simulink library "DBX_model"  (R2015a)
settings: Solver=ode45  SolverMode=SingleTasking  StartTime=0.0  StopTime=10.0  RelTol=1e-3
undefined symbols (not defined in the file): a, A_M, Activo, C_d0, Ganancia, h, h_1, h_3, Initial_Omegas, Initial_Torques, J_T, kappa_Q, kappa_T, l, L_M, lambda_0_Q, lambda_0_T, Motor, Newton, Prop, R, Raphson, rho, Rotation_sign, sigma, Tau_motors, theta_0, theta_1, Throtle_TTO_vec, Torque_TTO_vec, trim_control, v_i0, v_i_adim, Vx_adim, Vz_adim
libraries: vrlib x11, DBX_model x9, simulink x3, aerolibutil x3, dspinverses x1
settings Model: Creator=David  LastModifiedBy=david
settings OptimizationCC: BlockReduction=off  BooleanDataType=off
settings DebuggingCC: SaveWithParameterizedLinksMsg=none  UnderspecifiedInitializationDetection=Classic  MergeDetectMultiDrivingBlocksExec=none  SignalResolutionControl=TryResolveAllWithWarning  StrictBusMsg=Warning
settings HardwareCC: TargetUnknown=on

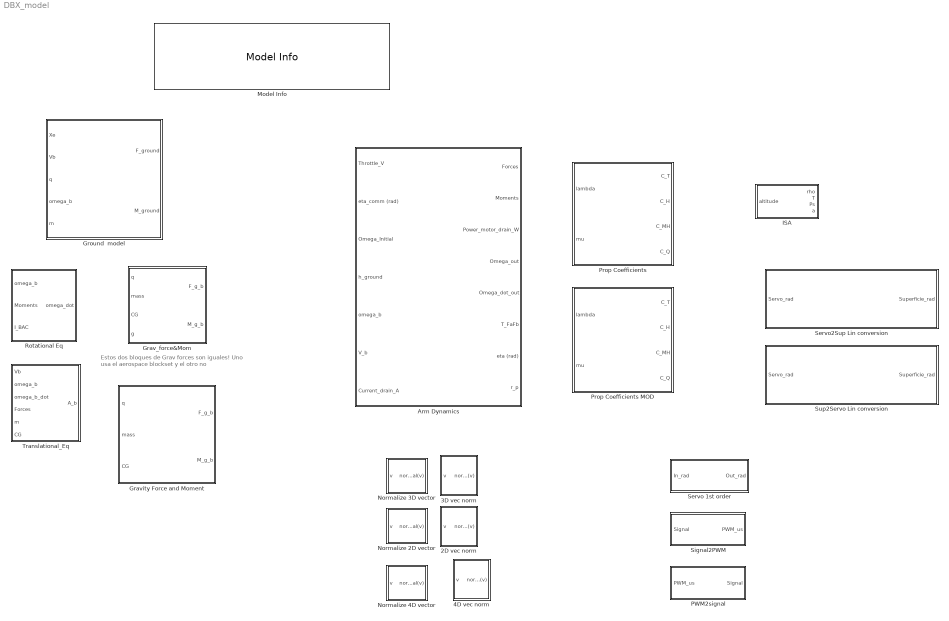
== system DBX_model ==
  note: Estos dos bloques de Grav forces son iguales!
      | Uno usa el aerospace blockset y el otro no
  2D vec norm : Subsystem
  3D vec norm : Subsystem
  4D vec norm : Subsystem
  Arm Dynamics : Subsystem  mask(Arm dynamics, kinematics, forces and moments){arm_num=1, Rot_sign=Rotation_sign(1), Hub_pos=l*[1;0;0], h_p=h, Gain=[1;0;0], UpperLimit=deg2rad(10), LowerLimit=-deg2rad(100), J_FA=0, Inertia_swithc_var=Motor+Prop, Freno_param=Activo, J_T=J_T, tau=Tau_motors, Initi_omega=Initial_Omegas(1), Init_torque=Initial_Torques(1), omega_n=35, xi=1.45, init_eta=0, Gain_servos=1, Bias=0.0}
      mask prompts: arm_num "Arm number (1,2 or 3)"; Rot_sign "Rotation sign"; Hub_pos "Hub position"; h_p "Hub to porpeller dist"; Gain "eta dir"; UpperLimit "eta sup lim"; LowerLimit "eta inf lim"; J_FA "J Fore arm"; Inertia_swithc_var "Which inertia to use?"; Freno_param "Freando o Activo"; J_T "Inertia Motor+Prop"; tau "Tau motors"; Initi_omega "Initial Omega (rad/s)"; Init_torque "Initial Torque(Nm)"; omega_n "Servo natural freq (rad/s) omega_n"; xi "Servo damping xi"; init_eta "Initial eta_servo (rad)"; Gain_servos "Pendiente Sup_rad/Servo_rad"; Bias "Sup_rad_0: Deflexion superficie con servo en 1500us"
      mask help:
      | This block only accepts arms oriented in x-axis or y-axis: eta direction can only be [1,0,0] or [0,1,0]
      |
      | If Arm number 1 or  2 (Forward ones)
      | eta_dir==[0,1,0]
      |
      | If Arm number 3 (rear one)
      | eta_dir=[1,0,0]
      |
      | Usar SIEMPRE SI
      mask TypeOptions arm_num: Arms Kinematics DBX/Value
      mask TypeOptions Rot_sign: Gyroscopic Moments DBX/Rot_sign | Aerodynamics Propeller DBX/Rot_signa
      mask TypeOptions Hub_pos: Arms Kinematics DBX/Hub_pos
      mask TypeOptions h_p: Arms Kinematics DBX/h_p
      mask TypeOptions Gain: Arms Kinematics DBX/Gain | Gyroscopic Moments DBX/Gain
      mask TypeOptions UpperLimit: Servos Dynamics DBX/UpperLimit
      mask TypeOptions LowerLimit: Servos Dynamics DBX/LowerLimit
      mask TypeOptions J_FA: Gyroscopic Moments DBX/J_FA
      mask TypeOptions Inertia_swithc_var: ESC+Motor Dynamcis DBX/Inertia_swithc_var
      mask TypeOptions Freno_param: ESC+Motor Dynamcis DBX/Freno_param
      mask TypeOptions J_T: ESC+Motor Dynamcis DBX/J_T | Gyroscopic Moments DBX/J_T
      mask TypeOptions tau: ESC+Motor Dynamcis DBX/tau
      mask TypeOptions Initi_omega: initial_omega/X0
      mask TypeOptions Init_torque: Initial_torque/X0
      mask TypeOptions omega_n: Servos Dynamics DBX/omega_n
      mask TypeOptions xi: Servos Dynamics DBX/xi | Servos Dynamics DBX/derv_param
      mask TypeOptions init_eta: Servos Dynamics DBX/init_eta
      mask TypeOptions Gain_servos: Servo2Sup Lin conversion/Gain
      mask TypeOptions Bias: Servo2Sup Lin conversion/Bias
      mask Display: disp(['{\bf \fontsize{16}',sprintf('Arm number\n\n'),num2str(arm_num),sprintf('\n\n Dynamics '),'}'], 'texmode','on');
  Grav_force&Mom : Subsystem
  Gravity Force and Moment : MATLAB Function
  Ground  model : Subsystem
  ISA : MATLAB Function  TreatAsAtomicUnit=on
  Model Info : simulink/Model-Wide Utilities/Model Info  Frame=on  DisplayStringWithTags=|  HorizontalTextAlignment=Center  LeftAlignmentValue=0.5  SourceBlockDiagram=DBX_model  TagMaxNumber=20
      | Model Info
      | 
      | Creado por %<Creator>
      | Modificado el %<LastModificationDate> por %<LastModifiedBy>
      | Version %<ModelVersion>
  Normalize 2D vector : Subsystem
  Normalize 3D vector : Subsystem
  Normalize 4D vector : Subsystem
  PWM2signal : Subsystem  TreatAsAtomicUnit=on  mask{c=1900, a=1100, d=1, b=0}
      mask prompts: c "PWM sup limit (us)"; a "PWM inf limit (us)"; d "Signal sup limit"; b "Signal inf limit"
      mask TypeOptions c: up_PWM/Value
      mask TypeOptions a: down_PWM/Value
      mask TypeOptions d: up_signal/Value
      mask TypeOptions b: down_signal/Value
  Prop Coefficients : MATLAB Function
  Prop Coefficients MOD : MATLAB Function
  Rotational Eq : Subsystem
  Servo 1st order : Subsystem  TreatAsAtomicUnit=on  mask{Init_def=0, Max_rate=6.159, Min_rate=-6.159, Max_defle=deg2rad(25), Min_def=-deg2rad(25), RT=0.01}
      mask prompts: Init_def "Initial deflection (rad)"; Max_rate "Maximo rate (rad/s)"; Min_rate "Minimo rate (rad/s)"; Max_defle "Maxima deflexion (rad)"; Min_def "Minima deflexion (rad)"; RT "Rise Time"
      mask TypeOptions Init_def: Initial/Value
      mask TypeOptions Max_rate:
      | Rate
      | Saturation/UpperLimit
      mask TypeOptions Min_rate:
      | Rate
      | Saturation/LowerLimit
      mask TypeOptions Max_defle:
      | Command
      | Saturation/UpperLimit | Integrator
      | /UpperSaturationLimit
      mask TypeOptions Min_def:
      | Command
      | Saturation/LowerLimit | Integrator
      | /LowerSaturationLimit
      mask Callback RT:
      | vals=get_param(gcb,'MaskValues');
      | Ganancia = 1/str2num(vals{6});
  Servo2Sup Lin conversion : Subsystem  mask{Gain=1, Bias=0.0}
      mask prompts: Gain "Pendiente Sup_rad/Servo_rad"; Bias "Sup_rad_0: Deflexion superficie con servo en 1500us"
      mask TypeOptions Gain: Gain/Gain
      mask TypeOptions Bias: Bias/Bias
      mask DialogControl DescTextVar Prompt: Conversion de roation del servo en rad a deflexion de las superficie de control en rad. Usar la funcion de matlab para encontrar las variables de abajo
      mask Display:
      | x=-pi:0.1:pi;
      | y=Gain.*x+Bias;
      | 
      | plot(x,y);
      | 
      | 
      | port_label('output', 1, 'Defl Superficie rad')
      | 
      | port_label('input', 1, 'Rotacion servo rad')
  Signal2PWM : Subsystem  TreatAsAtomicUnit=on  mask{b=1, d=0, a=1900, c=1100}
      mask prompts: b "Signal sup limit"; d "Signal inf limit"; a "PWM sup limit (us)"; c "PWM inf limit (us)"
      mask TypeOptions b: up_signal/Value
      mask TypeOptions d: down_signal/Value
      mask TypeOptions a: up_PWM/Value
      mask TypeOptions c: down_PWM/Value
  Sup2Servo Lin conversion : Subsystem  mask{Gain=1, Bias=0.0}
      mask prompts: Gain "Pendiente Sup_rad/Servo_rad"; Bias "Sup_rad_0: Deflexion superficie con servo en 1500us"
      mask TypeOptions Gain: Sup to servo pendiente/Value
      mask TypeOptions Bias: Sup_0_rad/Value
      mask DialogControl DescTextVar Prompt: Conversion de deflexion de la superficie en rad a rotacion del servo en rad. Usar la funcion de matlab para encontrar las variables de abajo
      mask Display:
      | x=-pi:0.1:pi;
      | y=(x-Bias)./Gain;
      | 
      | plot(x,y);
      | 
      | port_label('output', 1, 'Rotacion servo rad')
      | port_label('input', 1, 'Defl Superficie rad')
  Translational_Eq : Subsystem

== system DBX_model/2D vec norm ==
  v : Inport
  norm^2rm : Subsystem  TreatAsAtomicUnit=on
  sqrt : Sqrt  AlgorithmType=Newton-Raphson  SaturateOnIntegerOverflow=on
  norm(v) : Outport
  wires:
  sqrt/1 -> norm(v)/1
  norm^2rm/1(norm(v)) -> sqrt/1
  v/1 -> norm^2rm/1(v)

== system DBX_model/3D vec norm ==
  v : Inport
  norm^2rm : Subsystem  TreatAsAtomicUnit=on
  sqrt : Sqrt  AlgorithmType=Newton-Raphson  SaturateOnIntegerOverflow=on
  norm(v) : Outport
  wires:
  v/1 -> norm^2rm/1(v)
  norm^2rm/1(norm(v)) -> sqrt/1
  sqrt/1 -> norm(v)/1

== system DBX_model/4D vec norm ==
  v : Inport
  norm^2rm : Subsystem  TreatAsAtomicUnit=on
  sqrt : Sqrt  AlgorithmType=Newton-Raphson  SaturateOnIntegerOverflow=on
  norm(v) : Outport
  wires:
  sqrt/1 -> norm(v)/1
  norm^2rm/1(norm(v)) -> sqrt/1
  v/1 -> norm^2rm/1(v)

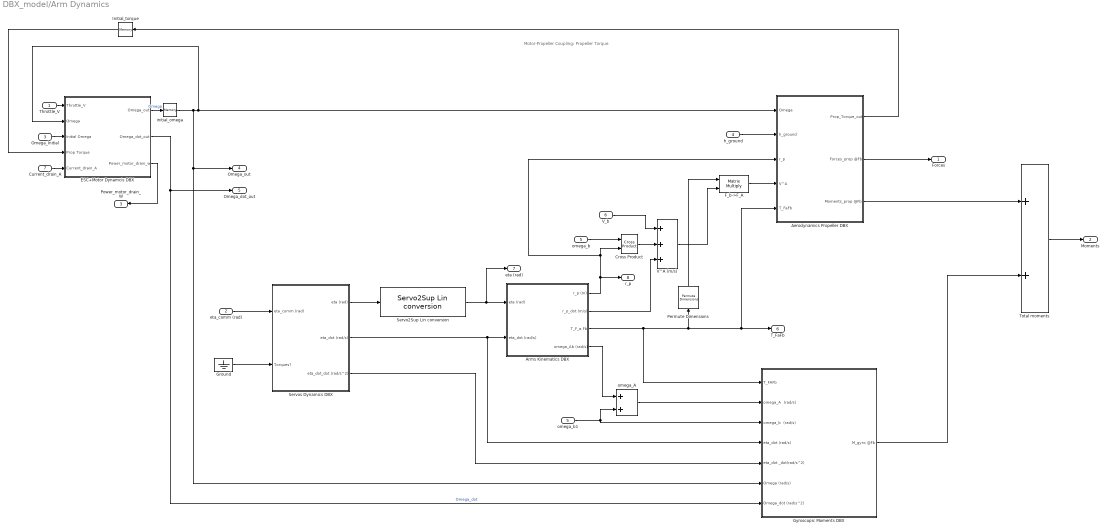
== system DBX_model/Arm Dynamics ==
  note: Motor-Propeller Coupling: Propeller Torque
  Throttle_V : Inport
  eta_comm (rad) : Inport  Port=2
  Omega_Initial : Inport  Port=3
  h_ground : Inport  Port=4
  omega_b : Inport  Port=5
  V_b : Inport  Port=6
  Current_drain_A : Inport  Port=7
  Aerodynamics Propeller DBX : Subsystem  mask{Rot_signa=Rot_sign}
      mask prompts: Rot_signa "Rotation Sign"
      settings: MinAlgLoopOccurrences=on
      mask TypeOptions Rot_signa: Rotation_sign/Value
  Arms Kinematics DBX : Subsystem  mask{Value=arm_num, Hub_pos=Hub_pos, h_p=h_p, Gain=Gain}
      mask prompts: Value "Arm number (1,2 or 3)"; Hub_pos "Hub position"; h_p "Hub to porpeller dist"; Gain "eta dir"
      mask TypeOptions Value: Arm_no/Value
      mask TypeOptions Hub_pos: Hub_position aka r_RP_i/Value
      mask TypeOptions h_p: h_p_i/Value
      mask TypeOptions Gain: eta_dir/Gain
  Cross Product : vrlib/Utilities/Cross Product
  ESC+Motor Dynamcis DBX : Subsystem  mask{Inertia_swithc_var=Motor+Prop, J_T=J_T, tau=tau, Freno_param=Activo}
      mask prompts: Inertia_swithc_var "Which inertia to use?"; J_T "Inertia Motor+Prop"; tau "Tau motors"; Freno_param "Freando o Activo"
      mask init:
      | val = get_param(gcb,'MaskValues');
      | switch lower(val{4})
      |  case {'frenado'}
      |   Freno=0;
      |  case {'activo'}
      |   Freno=1;
      | end
      mask TypeOptions Inertia_swithc_var: None | Motor+Prop
      mask Callback Inertia_swithc_var:
      | val = get_param(gcb,'MaskValues');
      | % lower(val{1})
      | switch lower(val{1})
      |  case {'none'}
      |   inertia_switch=1;
      |  case {'motor+prop'}
      |   inertia_switch=2;
      | end
      mask TypeOptions J_T: Inertia of prop+motor/Value
      mask TypeOptions tau: Time constant motors/Value
      mask TypeOptions Freno_param: Frenado | Activo
      mask Callback Freno_param:
      | val = get_param(gcb,'MaskValues');
      | switch lower(val{4})
      |  case {'frenado'}
      |   Freno=0;
      |  case {'activo'}
      |   Freno=1;
      | end
  F_b->F_A : Product  Multiplication=Matrix(*)
  Ground : Ground
  Gyroscopic Moments DBX : Subsystem  mask{Rot_sign=Rot_sign, Gain=Gain, J_T=J_T, J_FA=J_FA}
      mask prompts: Rot_sign "Rotation sign"; Gain "eta direction"; J_T "Motor&prop inertia"; J_FA "J Fore arm"
      mask TypeOptions Rot_sign: Rotation_sign/Value | Rotation_sign1/Value
      mask TypeOptions Gain: eta_dir/Gain | eta_dir1/Gain
      mask TypeOptions J_T: Propeller and motor inertia1/Value | Propeller and motor inertia/Value
  Initial_torque : Memory  X0=Init_torque  InheritSampleTime=on
  Permute Dimensions : PermuteDimensions
  Servo2Sup Lin conversion : DBX_model/Servo2Sup Lin conversion  Gain=Gain_servos  Bias=Bias
  Servos Dynamics DBX : Subsystem  mask{omega_n=omega_n, xi=xi, derv_param=xi, init_eta=init_eta, UpperLimit=UpperLimit, LowerLimit=LowerLimit, Gain=Gain_servos, Bias=Bias}
      mask prompts: omega_n "Servo natural freq (rad/s) omega_n"; xi "Servo damping xi"; derv_param "Derivative parameter"; init_eta "Initial eta_servo (rad)"; UpperLimit "eta Sup lim"; LowerLimit "eta inf lim"; Gain "Pendiente Sup_rad/Servo_rad"; Bias "Sup_rad_0: Deflexion superficie con servo en 1500us"
      mask TypeOptions init_eta: init_eta/Value | init_eta1/Value
      mask TypeOptions UpperLimit: upper limit/Value
      mask TypeOptions LowerLimit: Lower limit/Value
      mask TypeOptions Gain: Sup2Servo Lin conversion/Gain | Sup2Servo Lin conversion1/Gain
      mask TypeOptions Bias: Sup2Servo Lin conversion/Bias | Sup2Servo Lin conversion1/Bias
  Total moments : Sum
  V^A (m/s) : Sum  Inputs=+++
  initial_omega : Memory  X0=Initi_omega  InheritSampleTime=on
  omega_A : Sum
  omega_b1 : InportShadow  Port=5
  Forces : Outport
  Moments : Outport  Port=2
  Power_motor_drain_W : Outport  Port=3
  Omega_out : Outport  Port=4
  Omega_dot_out : Outport  Port=5
  T_FaFb : Outport  Port=6
  eta (rad) : Outport  Port=7
  r_p : Outport  Port=8
  wires:
  Throttle_V/1 -> ESC+Motor Dynamcis DBX/1(Throttle_V)
  Omega_Initial/1 -> ESC+Motor Dynamcis DBX/3(Initial Omega)
  ESC+Motor Dynamcis DBX/2(Omega_dot_out) -> Gyroscopic Moments DBX/7(Omega_dot (rad/s^2)), Omega_dot_out/1  "Omega_dot"
  ESC+Motor Dynamcis DBX/1(Omega_out) -> initial_omega/1  "Omega"
  h_ground/1 -> Aerodynamics Propeller DBX/2(h_ground)
  Servos Dynamics DBX/1(eta (rad)) -> Servo2Sup Lin conversion/1
  omega_b/1 -> Cross Product/1
  Cross Product/1 -> V^A (m/s)/2
  V_b/1 -> V^A (m/s)/1
  Arms Kinematics DBX/2(r_p_dot (m/s)) -> V^A (m/s)/3
  F_b->F_A/1 -> Aerodynamics Propeller DBX/4(V^A)
  Arms Kinematics DBX/3(T_F_a,Fb) -> Gyroscopic Moments DBX/1(T_FAFb), Permute Dimensions/1, Aerodynamics Propeller DBX/5(T_FaFb), T_FaFb/1
  Arms Kinematics DBX/1(r_p (m)) -> Aerodynamics Propeller DBX/3(r_p), Cross Product/2, r_p/1
  Aerodynamics Propeller DBX/2(Forces_prop @Fb) -> Forces/1
  Servos Dynamics DBX/2(eta_dot (rad/s)) -> Gyroscopic Moments DBX/4(eta_dot (rad/s)), Arms Kinematics DBX/2(eta_dot (rad/s))
  Arms Kinematics DBX/4(omega_Ab (rad/s)) -> omega_A/1
  omega_b1/1 -> Gyroscopic Moments DBX/3(omega_b  (rad/s)), omega_A/2
  omega_A/1 -> Gyroscopic Moments DBX/2(omega_A  (rad/s))
  Servos Dynamics DBX/3(eta_dot_dot (rad/s^2)) -> Gyroscopic Moments DBX/5(eta_dot _dot(rad/s^2))
  Ground/1 -> Servos Dynamics DBX/2(Torques?)
  Aerodynamics Propeller DBX/3(Moments_prop @Fb) -> Total moments/1
  Gyroscopic Moments DBX/1(M_gyro @Fb) -> Total moments/2
  Total moments/1 -> Moments/1
  Aerodynamics Propeller DBX/1(Prop_Torque_out) -> Initial_torque/1
  Initial_torque/1 -> ESC+Motor Dynamcis DBX/4(Prop Torque)
  eta_comm (rad)/1 -> Servos Dynamics DBX/1(eta_comm (rad))
  Servo2Sup Lin conversion/1 -> Arms Kinematics DBX/1(eta (rad)), eta (rad)/1
  V^A (m/s)/1 -> F_b->F_A/2
  Permute Dimensions/1 -> F_b->F_A/1
  initial_omega/1 -> Aerodynamics Propeller DBX/1(Omega), ESC+Motor Dynamcis DBX/2(Omega), Gyroscopic Moments DBX/6(Omega (rad/s)), Omega_out/1
  ESC+Motor Dynamcis DBX/3(Power_motor_drain_w) -> Power_motor_drain_W/1
  Current_drain_A/1 -> ESC+Motor Dynamcis DBX/5(Current_drain_A)

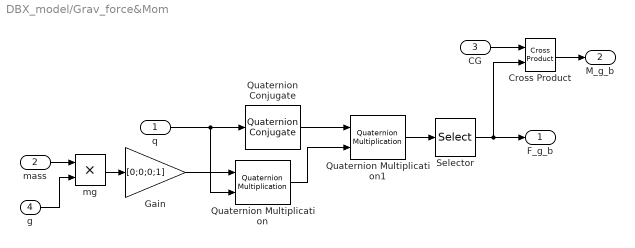
== system DBX_model/Grav_force&Mom ==
  q : Inport
  mass : Inport  Port=2
  CG : Inport  Port=3
  g : Inport  Port=4
  Cross Product : vrlib/Utilities/Cross Product
  Gain : Gain  Gain=[0;0;0;1]
  Quaternion Conjugate : aerolibutil/Quaternion Conjugate
  Quaternion Multiplication : aerolibutil/Quaternion Multiplication
  Quaternion Multiplication1 : aerolibutil/Quaternion Multiplication
  Selector : Selector  IndexMode=Zero-based  InputPortWidth=4  Indices=[1:3]
  mg : Product  RndMeth=Zero
  F_g_b : Outport
  M_g_b : Outport  Port=2
  wires:
  mass/1 -> mg/1
  g/1 -> mg/2
  mg/1 -> Gain/1
  Gain/1 -> Quaternion Multiplication/1
  q/1 -> Quaternion Conjugate/1, Quaternion Multiplication/2
  Quaternion Conjugate/1 -> Quaternion Multiplication1/1
  Quaternion Multiplication/1 -> Quaternion Multiplication1/2
  Quaternion Multiplication1/1 -> Selector/1
  Selector/1 -> Cross Product/2, F_g_b/1
  CG/1 -> Cross Product/1
  Cross Product/1 -> M_g_b/1

== system DBX_model/Ground  model ==
  Xe : Inport
  Vb : Inport  Port=2
  q : Inport  Port=3
  omega_b : Inport  Port=4
  m : Inport  Port=5
  Ground model logic and Forces and moments : MATLAB Function  TreatAsAtomicUnit=on
  arm_hub position 1 : Constant  Value=[1/3*L_M;-A_M/2;h_1]
  arm_hub position 2 : Constant  Value=[1/3*L_M;A_M/2;h_1]
  arm_hub position 3 : Constant  Value=[-2/3*L_M;0;h_3]
  F_ground : Outport
  M_ground : Outport  Port=2
  wires:
  omega_b/1 -> Ground model logic and Forces and moments/4(omega_b)
  Vb/1 -> Ground model logic and Forces and moments/2(Vb)
  Ground model logic and Forces and moments/1(F_gr_b) -> F_ground/1
  Ground model logic and Forces and moments/2(M_gr_b) -> M_ground/1
  arm_hub position 3/1 -> Ground model logic and Forces and moments/8(Arm3)
  arm_hub position 2/1 -> Ground model logic and Forces and moments/7(Arm2)
  arm_hub position 1/1 -> Ground model logic and Forces and moments/6(Arm1)
  m/1 -> Ground model logic and Forces and moments/5(mass)
  q/1 -> Ground model logic and Forces and moments/3(q)
  Xe/1 -> Ground model logic and Forces and moments/1(Xe)

== system DBX_model/Normalize 2D vector ==
  v : Inport
  2D vec norm : DBX_model/2D vec norm
  Bias : Bias  Bias=eps
  Demux : Demux  Outputs=2
  Math Function : Math  Operator=reciprocal  SaturateOnIntegerOverflow=on
  Mux : Mux  Inputs=2
  Product2 : Product  Inputs=**
  Product3 : Product  Inputs=**
  normal(v) : Outport
  wires:
  Math Function/1 -> Product2/2, Product3/2
  Demux/2 -> Product3/1
  Demux/1 -> Product2/1
  Mux/1 -> normal(v)/1
  v/1 -> 2D vec norm/1, Demux/1
  Bias/1 -> Math Function/1
  Product2/1 -> Mux/1
  Product3/1 -> Mux/2
  2D vec norm/1 -> Bias/1

== system DBX_model/Normalize 3D vector ==
  v : Inport
  3D vec norm : DBX_model/3D vec norm
  Bias : Bias  Bias=eps
  Demux : Demux  Outputs=3
  Math Function : Math  Operator=reciprocal  SaturateOnIntegerOverflow=on
  Mux : Mux  Inputs=3
  Product1 : Product  Inputs=**
  Product2 : Product  Inputs=**
  Product3 : Product  Inputs=**
  normal(v) : Outport
  wires:
  Demux/2 -> Product3/1
  Demux/1 -> Product2/1
  Mux/1 -> normal(v)/1
  v/1 -> 3D vec norm/1, Demux/1
  3D vec norm/1 -> Bias/1
  Product2/1 -> Mux/1
  Product3/1 -> Mux/2
  Demux/3 -> Product1/1
  Math Function/1 -> Product2/2, Product3/2, Product1/2
  Product1/1 -> Mux/3
  Bias/1 -> Math Function/1

== system DBX_model/Normalize 4D vector ==
  v : Inport
  4D vec norm : DBX_model/4D vec norm
  Bias : Bias  Bias=eps
  Demux : Demux
  Math Function : Math  Operator=reciprocal  SaturateOnIntegerOverflow=on
  Mux : Mux
  Product{1..4} (4 alike) : Product  Inputs=**
  normal(v) : Outport
  wires:
  Product4/1 -> Mux/4
  Demux/4 -> Product4/1
  Demux/2 -> Product3/1
  Demux/1 -> Product2/1
  Mux/1 -> normal(v)/1
  v/1 -> 4D vec norm/1, Demux/1
  4D vec norm/1 -> Bias/1
  Product2/1 -> Mux/1
  Product3/1 -> Mux/2
  Demux/3 -> Product1/1
  Math Function/1 -> Product2/2, Product3/2, Product1/2, Product4/2
  Product1/1 -> Mux/3
  Bias/1 -> Math Function/1

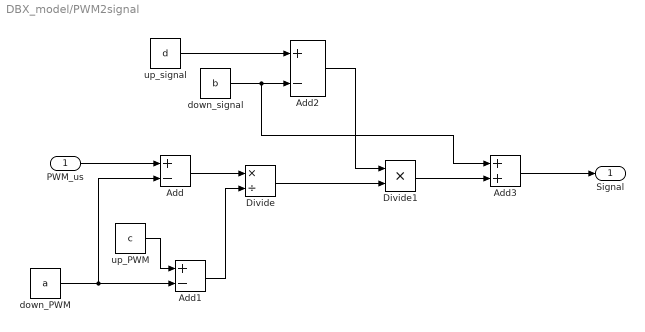
== system DBX_model/PWM2signal ==
  PWM_us : Inport
  Add : Sum  Inputs=+-
  Add1 : Sum  Inputs=+-
  Add2 : Sum  Inputs=+-
  Add3 : Sum
  Divide : Product  Inputs=*/
  Divide1 : Product  Inputs=**
  down_PWM : Constant  Value=a
  down_signal : Constant  Value=b
  up_PWM : Constant  Value=c
  up_signal : Constant  Value=d
  Signal : Outport
  wires:
  PWM_us/1 -> Add/1
  down_PWM/1 -> Add/2, Add1/2
  up_PWM/1 -> Add1/1
  Add1/1 -> Divide/2
  Add/1 -> Divide/1
  up_signal/1 -> Add2/1
  down_signal/1 -> Add3/1, Add2/2
  Divide/1 -> Divide1/2
  Add2/1 -> Divide1/1
  Divide1/1 -> Add3/2
  Add3/1 -> Signal/1

== system DBX_model/Rotational Eq ==
  omega_b : Inport
  Moments : Inport  Port=2
  I_BAC : Inport  Port=3
  " LU Inverse" : dspinverses/ LU Inverse
  Add : Sum  Inputs=+-
  Cross Product : vrlib/Utilities/Cross Product
  Gain : Gain  Gain=-1
  Matrix Multiply : Product  Multiplication=Matrix(*)
  Matrix Multiply1 : Product  Multiplication=Matrix(*)
  omega_dot : Outport
  wires:
  I_BAC/1 -> " LU Inverse"/1, Matrix Multiply/1
  omega_b/1 -> Cross Product/1, Matrix Multiply/2
  Matrix Multiply/1 -> Cross Product/2
  Cross Product/1 -> Gain/1
  Moments/1 -> Add/1
  Gain/1 -> Add/2
  Add/1 -> Matrix Multiply1/2
  " LU Inverse"/1 -> Matrix Multiply1/1
  Matrix Multiply1/1 -> omega_dot/1

== system DBX_model/Servo 1st order ==
  In_rad : Inport
  Command Saturation : Saturate  UpperLimit=Max_defle  LowerLimit=Min_def
  Gain : Gain  Gain=Ganancia  SaturateOnIntegerOverflow=on  OutDataTypeStr=Inherit: Same as input  ParamDataTypeStr=Inherit: Same as input
  Initial : Constant  Value=Init_def
  "Integrator " : Integrator  InitialConditionSource=external  InitialCondition=trim_control(2)  LimitOutput=on  UpperSaturationLimit=Max_defle  LowerSaturationLimit=Min_def
  Rate Saturation : Saturate  UpperLimit=Max_rate  LowerLimit=Min_rate
  Sum : Sum  Inputs=|+-  SaturateOnIntegerOverflow=on  InputSameDT=on  OutDataTypeStr=Inherit: Same as first input
  Out_rad : Outport
  wires:
  In_rad/1 -> Command Saturation/1
  Command Saturation/1 -> Sum/1
  Sum/1 -> Gain/1
  Gain/1 -> Rate Saturation/1
  Rate Saturation/1 -> "Integrator "/1
  "Integrator "/1 -> Out_rad/1, Sum/2
  Initial/1 -> "Integrator "/2

== system DBX_model/Servo2Sup Lin conversion ==
  Servo_rad : Inport
  Bias : Bias  Bias=Bias
  Gain : Gain  Gain=Gain
  Superficie_rad : Outport
  wires:
  Gain/1 -> Bias/1
  Servo_rad/1 -> Gain/1
  Bias/1 -> Superficie_rad/1

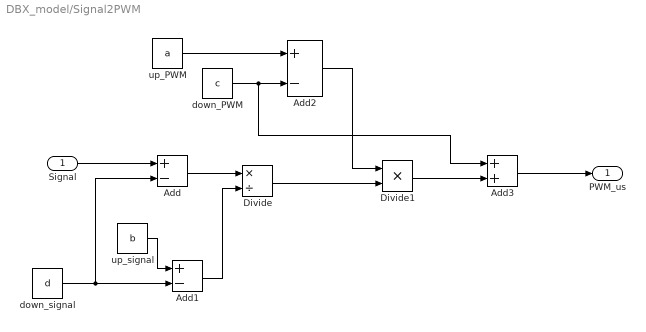
== system DBX_model/Signal2PWM ==
  Signal : Inport
  Add : Sum  Inputs=+-
  Add1 : Sum  Inputs=+-
  Add2 : Sum  Inputs=+-
  Add3 : Sum  OutDataTypeStr=int32
  Divide : Product  Inputs=*/
  Divide1 : Product  Inputs=**
  down_PWM : Constant  Value=c
  down_signal : Constant  Value=d
  up_PWM : Constant  Value=a
  up_signal : Constant  Value=b
  PWM_us : Outport  OutDataTypeStr=int32
  wires:
  Add3/1 -> PWM_us/1
  Divide1/1 -> Add3/2
  Add2/1 -> Divide1/1
  Divide/1 -> Divide1/2
  down_PWM/1 -> Add2/2, Add3/1
  up_PWM/1 -> Add2/1
  Add/1 -> Divide/1
  Add1/1 -> Divide/2
  up_signal/1 -> Add1/1
  down_signal/1 -> Add1/2, Add/2
  Signal/1 -> Add/1

== system DBX_model/Sup2Servo Lin conversion ==
  Servo_rad : Inport
  Divide : Product  Inputs=*/
  Subtract : Sum  Inputs=+-
  Sup to servo pendiente : Constant  Value=Gain
  Sup_0_rad : Constant  Value=Bias
  Superficie_rad : Outport
  wires:
  Servo_rad/1 -> Subtract/1
  Sup_0_rad/1 -> Subtract/2
  Subtract/1 -> Divide/1
  Sup to servo pendiente/1 -> Divide/2
  Divide/1 -> Superficie_rad/1

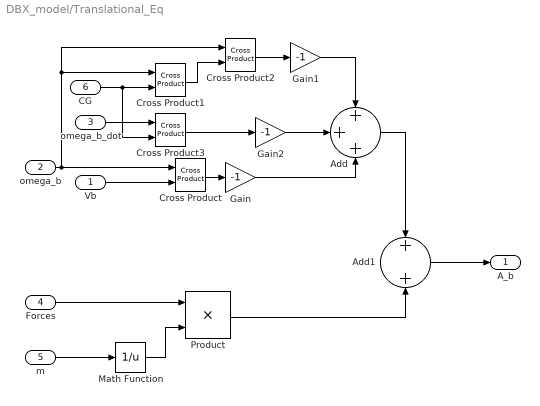
== system DBX_model/Translational_Eq ==
  Vb : Inport
  omega_b : Inport  Port=2
  omega_b_dot : Inport  Port=3
  Forces : Inport  Port=4
  m : Inport  Port=5
  CG : Inport  Port=6
  Add : Sum  Inputs=+++
  Add1 : Sum
  Cross Product{,1..3} (4 alike) : vrlib/Utilities/Cross Product
  Gain : Gain  Gain=-1
  Gain1 : Gain  Gain=-1
  Gain2 : Gain  Gain=-1
  Math Function : Math  Operator=reciprocal  SaturateOnIntegerOverflow=on
  Product : Product  RndMeth=Zero
  A_b : Outport
  wires:
  m/1 -> Math Function/1
  Math Function/1 -> Product/2
  Forces/1 -> Product/1
  omega_b/1 -> Cross Product2/1, Cross Product1/1, Cross Product/1
  Vb/1 -> Cross Product/2
  Cross Product/1 -> Gain/1
  CG/1 -> Cross Product3/2, Cross Product1/2
  Cross Product1/1 -> Cross Product2/2
  Cross Product2/1 -> Gain1/1
  omega_b_dot/1 -> Cross Product3/1
  Cross Product3/1 -> Gain2/1
  Gain1/1 -> Add/1
  Gain2/1 -> Add/2
  Gain/1 -> Add/3
  Product/1 -> Add1/2
  Add/1 -> Add1/1
  Add1/1 -> A_b/1

== system DBX_model/2D vec norm/norm^2rm ==
  v : Inport
  Demux : Demux  Outputs=2
  Product : Product
  Product1 : Product
  Sum : Sum  Inputs=2
  norm(v) : Outport
  wires:
  v/1 -> Demux/1
  Sum/1 -> norm(v)/1
  Product/1 -> Sum/1
  Product1/1 -> Sum/2
  Demux/1 -> Product/1, Product/2
  Demux/2 -> Product1/2, Product1/1

== system DBX_model/3D vec norm/norm^2rm ==
  v : Inport
  Demux : Demux  Outputs=3
  Product : Product
  Product1 : Product
  Product2 : Product
  Sum : Sum  Inputs=3
  norm(v) : Outport
  wires:
  Demux/2 -> Product1/2, Product1/1
  Demux/1 -> Product/2, Product/1
  Product1/1 -> Sum/2
  Product/1 -> Sum/1
  Sum/1 -> norm(v)/1
  v/1 -> Demux/1
  Demux/3 -> Product2/2, Product2/1
  Product2/1 -> Sum/3

== system DBX_model/4D vec norm/norm^2rm ==
  v : Inport
  Demux : Demux
  Product{,1..3} (4 alike) : Product
  Sum : Sum  Inputs=4
  norm(v) : Outport
  wires:
  Product3/1 -> Sum/4
  Demux/4 -> Product3/1, Product3/2
  Product2/1 -> Sum/3
  Demux/3 -> Product2/1, Product2/2
  v/1 -> Demux/1
  Sum/1 -> norm(v)/1
  Product/1 -> Sum/1
  Product1/1 -> Sum/2
  Demux/1 -> Product/1, Product/2
  Demux/2 -> Product1/1, Product1/2

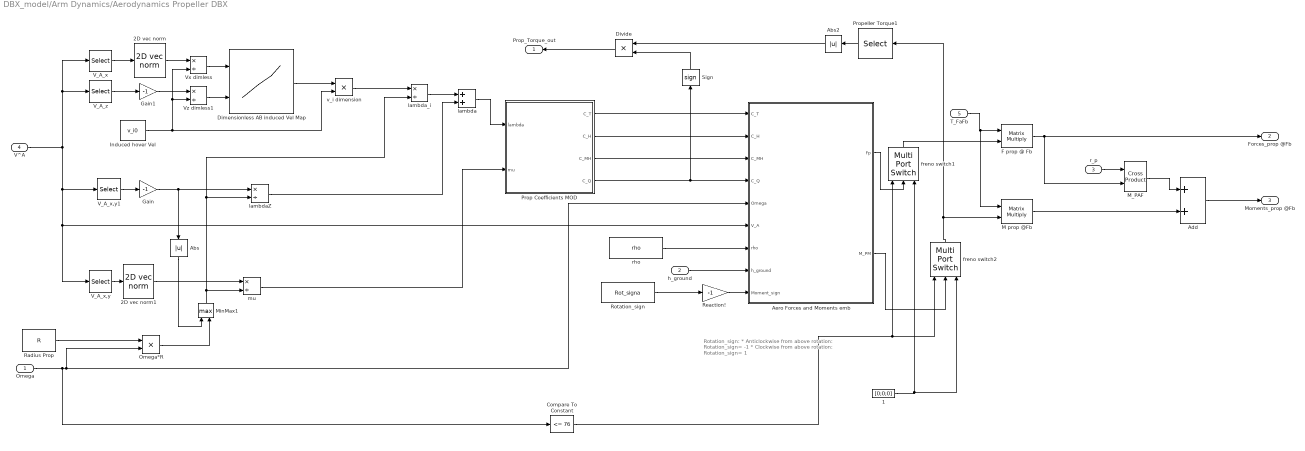
== system DBX_model/Arm Dynamics/Aerodynamics Propeller DBX ==
  note: Rotation_sign:
      |
      | * Anticlockwise from above rotation: Rotation_sign= -1
      | * Clockwise from above rotation: Rotation_sign= 1
  Omega : Inport
  h_ground : Inport  Port=2
  r_p : Inport  Port=3
  V^A : Inport  Port=4
  T_FaFb : Inport  Port=5
  1 : Constant  Value=[0;0;0]
  2D vec norm : DBX_model/2D vec norm
  2D vec norm1 : DBX_model/2D vec norm
  Abs : Abs
  Abs2 : Abs
  Add : Sum
  Aero Forces and Moments emb : Subsystem
  Compare To Constant : simulink/Logic and Bit Operations/Compare To Constant  relop=<=  const=76  OutDataTypeStr=boolean
  Dimensionless AB induced Vel Map : Lookup_n-D  BreakpointsForDimension1=Vx_adim  BreakpointsForDimension2=Vz_adim  BreakpointsForDimension3=[5, 7]  Table=v_i_adim  RndMeth=Simplest  InputSameDT=on
  Divide : Product  Inputs=**
  F prop @ Fb : Product  Multiplication=Matrix(*)
  Gain : Gain  Gain=-1
  Gain1 : Gain  Gain=-1
  Induced hover Vel : Constant  Value=v_i0
  M prop @Fb : Product  Multiplication=Matrix(*)
  M_PAF : vrlib/Utilities/Cross Product
  MinMax1 : MinMax  Function=max  Inputs=2
  Omega*R : Product  Inputs=**
  Prop Coefficients MOD : MATLAB Function
  Propeller Torque1 : Selector  IndexMode=Zero-based  InputPortWidth=3  Indices=2
  Radius Prop : Constant  Value=R
  Reaction! : Gain  Gain=-1
  Rotation_sign : Constant  Value=Rot_signa
  Sign : Signum
  V_A_x : Selector  InputPortWidth=3  Indices=[1 2]
  V_A_x,y : Selector  InputPortWidth=3  Indices=[1 2]
  V_A_x,y1 : Selector  InputPortWidth=3  Indices=[3]
  V_A_z : Selector  InputPortWidth=3  Indices=3
  Vx dimless : Product  Inputs=*/
  Vz dimless1 : Product  Inputs=*/
  freno switch1 : MultiPortSwitch  DataPortOrder=Zero-based contiguous  Inputs=2
  freno switch2 : MultiPortSwitch  DataPortOrder=Zero-based contiguous  Inputs=2
  lambda : Sum
  lambdaZ : Product  Inputs=*/
  lambda_i : Product  Inputs=*/
  mu : Product  Inputs=*/
  rho : Constant  Value=rho
  v_i dimension : Product  Inputs=**
  Prop_Torque_out : Outport
  Forces_prop @Fb : Outport  Port=2
  Moments_prop @Fb : Outport  Port=3
  wires:
  Radius Prop/1 -> Omega*R/1
  V_A_x,y/1 -> 2D vec norm1/1
  2D vec norm1/1 -> mu/1
  Vx dimless/1 -> Dimensionless AB induced Vel Map/1
  V_A_x/1 -> 2D vec norm/1
  Vz dimless1/1 -> Dimensionless AB induced Vel Map/2
  V_A_z/1 -> Gain1/1
  Induced hover Vel/1 -> v_i dimension/2, Vz dimless1/2, Vx dimless/2
  Dimensionless AB induced Vel Map/1 -> v_i dimension/1
  v_i dimension/1 -> lambda_i/1
  V_A_x,y1/1 -> Gain/1
  Gain/1 -> lambdaZ/1, Abs/1
  lambda_i/1 -> lambda/1
  lambdaZ/1 -> lambda/2
  Gain1/1 -> Vz dimless1/1
  lambda/1 -> Prop Coefficients MOD/1(lambda)
  Prop Coefficients MOD/1(C_T) -> Aero Forces and Moments emb/1(C_T)
  Prop Coefficients MOD/2(C_H) -> Aero Forces and Moments emb/2(C_H)
  Prop Coefficients MOD/3(C_MH) -> Aero Forces and Moments emb/3(C_MH)
  V^A/1 -> V_A_x,y/1, Aero Forces and Moments emb/6(V_A), V_A_x,y1/1, V_A_x/1, V_A_z/1
  Add/1 -> Moments_prop @Fb/1
  h_ground/1 -> Aero Forces and Moments emb/8(h_ground)
  Rotation_sign/1 -> Reaction!/1
  T_FaFb/1 -> M prop @Fb/1, F prop @ Fb/1
  freno switch1/1 -> F prop @ Fb/2
  F prop @ Fb/1 -> M_PAF/2, Forces_prop @Fb/1
  r_p/1 -> M_PAF/1
  M_PAF/1 -> Add/1
  M prop @Fb/1 -> Add/2
  2D vec norm/1 -> Vx dimless/1
  mu/1 -> Prop Coefficients MOD/2(mu)
  Prop Coefficients MOD/4(C_Q) -> Sign/1, Aero Forces and Moments emb/4(C_Q)
  Reaction!/1 -> Aero Forces and Moments emb/9(Moment_sign)
  rho/1 -> Aero Forces and Moments emb/7(rho)
  Divide/1 -> Prop_Torque_out/1
  Propeller Torque1/1 -> Abs2/1
  Sign/1 -> Divide/2
  Abs2/1 -> Divide/1
  MinMax1/1 -> mu/2, lambdaZ/2, lambda_i/2
  Abs/1 -> MinMax1/1
  Omega*R/1 -> MinMax1/2
  Omega/1 -> Compare To Constant/1, Aero Forces and Moments emb/5(Omega), Omega*R/2
  freno switch2/1 -> Propeller Torque1/1, M prop @Fb/2
  Compare To Constant/1 -> freno switch1/1, freno switch2/1
  1/1 -> freno switch1/3, freno switch2/3
  Aero Forces and Moments emb/2("M_PM ") -> freno switch2/2
  Aero Forces and Moments emb/1(Fp) -> freno switch1/2

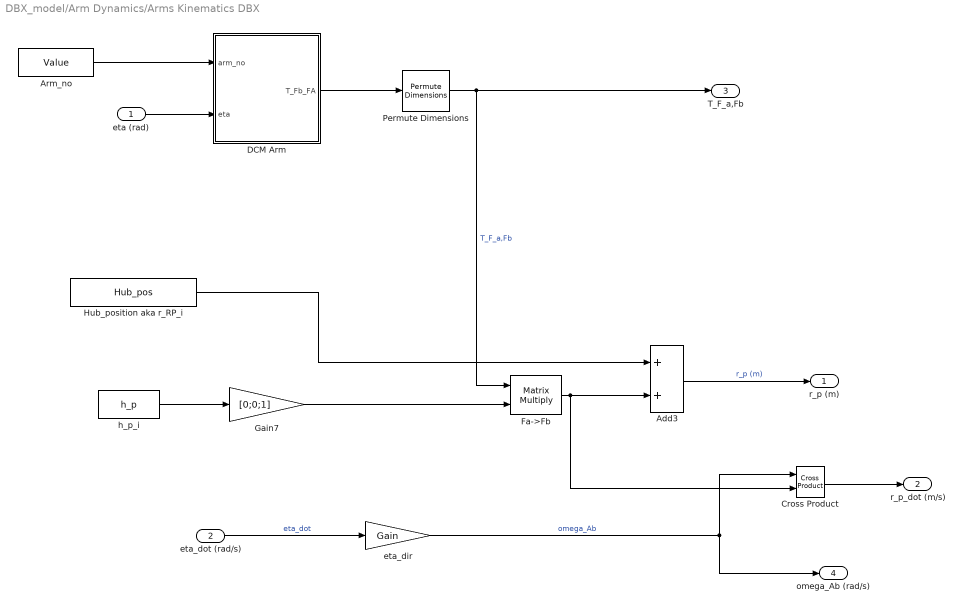
== system DBX_model/Arm Dynamics/Arms Kinematics DBX ==
  eta (rad) : Inport
  eta_dot (rad/s) : Inport  Port=2
  Add3 : Sum
  Arm_no : Constant  Value=Value
  Cross Product : vrlib/Utilities/Cross Product
  DCM Arm : MATLAB Function  TreatAsAtomicUnit=on
  Fa->Fb : Product  Multiplication=Matrix(*)
  Gain7 : Gain  Gain=[0;0;1]
  Hub_position aka r_RP_i : Constant  Value=Hub_pos
  Permute Dimensions : PermuteDimensions
  eta_dir : Gain  Gain=Gain
  h_p_i : Constant  Value=h_p
  r_p (m) : Outport
  r_p_dot (m/s) : Outport  Port=2
  T_F_a,Fb : Outport  Port=3
  omega_Ab (rad/s) : Outport  Port=4
  wires:
  Arm_no/1 -> DCM Arm/1(arm_no)
  Cross Product/1 -> r_p_dot (m/s)/1
  Fa->Fb/1 -> Add3/2, Cross Product/2
  Hub_position aka r_RP_i/1 -> Add3/1
  Gain7/1 -> Fa->Fb/2
  h_p_i/1 -> Gain7/1
  Add3/1 -> r_p (m)/1  "r_p (m)"
  eta_dir/1 -> omega_Ab (rad/s)/1, Cross Product/1  "omega_Ab"
  eta_dot (rad/s)/1 -> eta_dir/1  "eta_dot"
  eta (rad)/1 -> DCM Arm/2(eta)
  Permute Dimensions/1 -> Fa->Fb/1, T_F_a,Fb/1  "T_F_a,Fb"
  DCM Arm/1(T_Fb_FA) -> Permute Dimensions/1

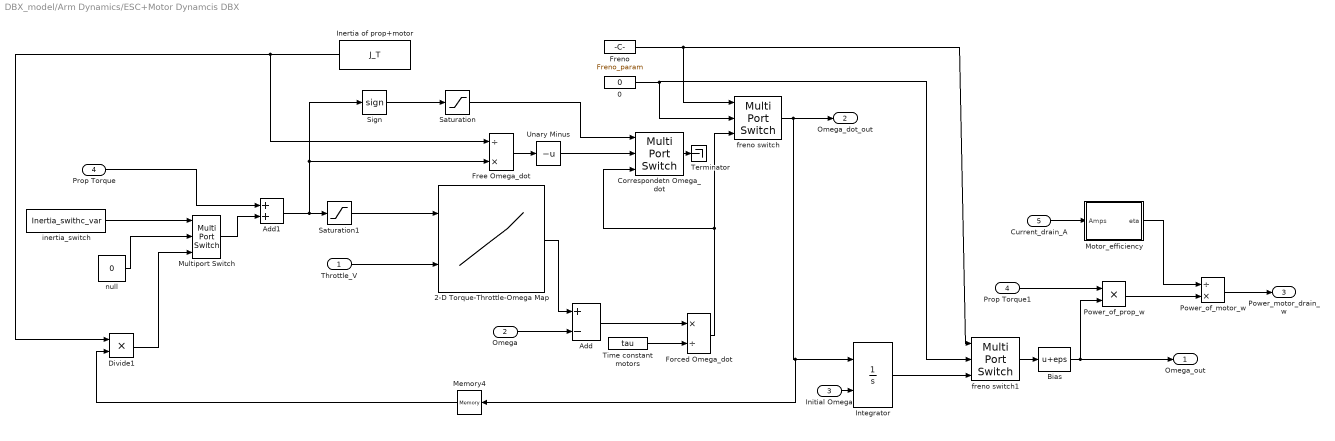
== system DBX_model/Arm Dynamics/ESC+Motor Dynamcis DBX ==
  Throttle_V : Inport
  Omega : Inport  Port=2
  Initial Omega : Inport  Port=3
  Prop Torque : Inport  Port=4
  Current_drain_A : Inport  Port=5
  0 : Constant  Value=0
  2-D Torque-Throttle-Omega Map : Lookup_n-D  BreakpointsForDimension1=Torque_TTO_vec  BreakpointsForDimension2=Throtle_TTO_vec  Table=Omega_TTO'  DiagnosticForOutOfRangeInput=Warning  RemoveProtectionInput=on  RndMeth=Simplest  InputSameDT=on
  Add : Sum  Inputs=+-
  Add1 : Sum
  Bias : Bias  Bias=eps
  Correspondetn Omega_dot : MultiPortSwitch  DataPortOrder=Zero-based contiguous  Inputs=2
  Divide1 : Product  Inputs=**
  Forced Omega_dot : Product  Inputs=*/
  Free Omega_dot : Product  Inputs=/*
  Freno : Constant  Value=Freno_param
  Inertia of prop+motor : Constant  Value=J_T
  Integrator : Integrator  InitialConditionSource=external
  Memory4 : Memory  InheritSampleTime=on
  Motor_efficiency : MATLAB Function  TreatAsAtomicUnit=on
  Multiport Switch : MultiPortSwitch  Inputs=2
  Power_of_motor_w : Product  Inputs=/*
  Power_of_prop_w : Product
  Prop Torque1 : InportShadow  Port=4
  Saturation : Saturate  UpperLimit=1  LowerLimit=0
  Saturation1 : Saturate  UpperLimit=inf  LowerLimit=0
  Sign : Signum
  Terminator : Terminator
  Time constant motors : Constant  Value=tau
  Unary Minus : UnaryMinus
  freno switch : MultiPortSwitch  Inputs=2
  freno switch1 : MultiPortSwitch  Inputs=2
  inertia_switch : Constant  Value=Inertia_swithc_var
  null : Constant  Value=0
  Omega_out : Outport
  Omega_dot_out : Outport  Port=2
  Power_motor_drain_w : Outport  Port=3
  wires:
  Unary Minus/1 -> Correspondetn Omega_dot/2
  Sign/1 -> Saturation/1
  Saturation/1 -> Correspondetn Omega_dot/1
  Free Omega_dot/1 -> Unary Minus/1
  Prop Torque/1 -> Add1/1
  2-D Torque-Throttle-Omega Map/1 -> Add/1
  Omega/1 -> Add/2
  Add/1 -> Forced Omega_dot/1
  Time constant motors/1 -> Forced Omega_dot/2
  Initial Omega/1 -> Integrator/2
  Multiport Switch/1 -> Add1/2
  Inertia of prop+motor/1 -> Divide1/1, Free Omega_dot/1
  null/1 -> Multiport Switch/2
  Throttle_V/1 -> 2-D Torque-Throttle-Omega Map/2
  freno switch/1 -> Memory4/1, Integrator/1, Omega_dot_out/1
  Memory4/1 -> Divide1/2
  inertia_switch/1 -> Multiport Switch/1
  Divide1/1 -> Multiport Switch/3
  Forced Omega_dot/1 -> Correspondetn Omega_dot/3, freno switch/3
  Freno/1 -> freno switch1/1, freno switch/1
  0/1 -> freno switch/2, freno switch1/2
  Integrator/1 -> freno switch1/3
  freno switch1/1 -> Bias/1
  Saturation1/1 -> 2-D Torque-Throttle-Omega Map/1
  Correspondetn Omega_dot/1 -> Terminator/1
  Add1/1 -> Saturation1/1, Free Omega_dot/2, Sign/1
  Bias/1 -> Power_of_prop_w/2, Omega_out/1
  Prop Torque1/1 -> Power_of_prop_w/1
  Power_of_prop_w/1 -> Power_of_motor_w/2
  Motor_efficiency/1(eta) -> Power_of_motor_w/1
  Power_of_motor_w/1 -> Power_motor_drain_w/1
  Current_drain_A/1 -> Motor_efficiency/1(Amps)

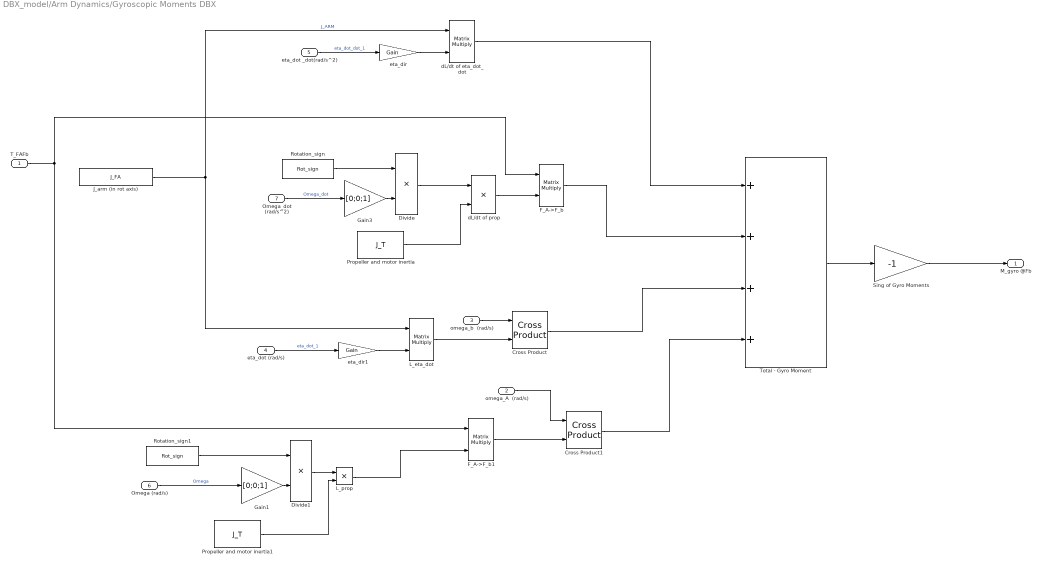
== system DBX_model/Arm Dynamics/Gyroscopic Moments DBX ==
  T_FAFb : Inport
  omega_A  (rad/s) : Inport  Port=2
  omega_b  (rad/s) : Inport  Port=3
  eta_dot (rad/s) : Inport  Port=4
  eta_dot _dot(rad/s^2) : Inport  Port=5
  Omega (rad/s) : Inport  Port=6
  Omega_dot (rad/s^2) : Inport  Port=7
  Cross Product : vrlib/Utilities/Cross Product
  Cross Product1 : vrlib/Utilities/Cross Product
  Divide : Product  Inputs=**
  Divide1 : Product  Inputs=**
  F_A->F_b : Product  Multiplication=Matrix(*)
  F_A->F_b1 : Product  Multiplication=Matrix(*)
  Gain1 : Gain  Gain=[0;0;1]
  Gain3 : Gain  Gain=[0;0;1]
  J_arm (in rot axis) : Constant  Value=J_FA
  L_eta_dot : Product  Multiplication=Matrix(*)
  L_prop : Product  Inputs=**
  Propeller and motor inertia : Constant  Value=J_T
  Propeller and motor inertia1 : Constant  Value=J_T
  Rotation_sign : Constant  Value=Rot_sign
  Rotation_sign1 : Constant  Value=Rot_sign
  Sing of Gyro Moments : Gain  Gain=-1
  Total - Gyro Moment : Sum  Inputs=++++
  dL/dt of eta_dot_dot : Product  Multiplication=Matrix(*)
  dL/dt of prop : Product  Inputs=**
  eta_dir : Gain  Gain=Gain
  eta_dir1 : Gain  Gain=Gain
  M_gyro @Fb : Outport
  wires:
  eta_dot _dot(rad/s^2)/1 -> eta_dir/1  "eta_dot_dot_1"
  J_arm (in rot axis)/1 -> L_eta_dot/1, dL/dt of eta_dot_dot/1  "J_ARM"
  eta_dir/1 -> dL/dt of eta_dot_dot/2
  eta_dir1/1 -> L_eta_dot/2
  eta_dot (rad/s)/1 -> eta_dir1/1  "eta_dot_1"
  L_eta_dot/1 -> Cross Product/2
  omega_b  (rad/s)/1 -> Cross Product/1
  Omega_dot (rad/s^2)/1 -> Gain3/1  "Omega_dot"
  Divide/1 -> dL/dt of prop/1
  Propeller and motor inertia/1 -> dL/dt of prop/2
  Divide1/1 -> L_prop/1
  Propeller and motor inertia1/1 -> L_prop/2
  Omega (rad/s)/1 -> Gain1/1  "Omega"
  dL/dt of prop/1 -> F_A->F_b/2
  F_A->F_b/1 -> Total - Gyro Moment/2
  dL/dt of eta_dot_dot/1 -> Total - Gyro Moment/1
  Cross Product/1 -> Total - Gyro Moment/3
  L_prop/1 -> F_A->F_b1/2
  T_FAFb/1 -> F_A->F_b/1, F_A->F_b1/1
  F_A->F_b1/1 -> Cross Product1/2
  omega_A  (rad/s)/1 -> Cross Product1/1
  Cross Product1/1 -> Total - Gyro Moment/4
  Total - Gyro Moment/1 -> Sing of Gyro Moments/1
  Sing of Gyro Moments/1 -> M_gyro @Fb/1
  Rotation_sign/1 -> Divide/1
  Gain3/1 -> Divide/2
  Rotation_sign1/1 -> Divide1/1
  Gain1/1 -> Divide1/2

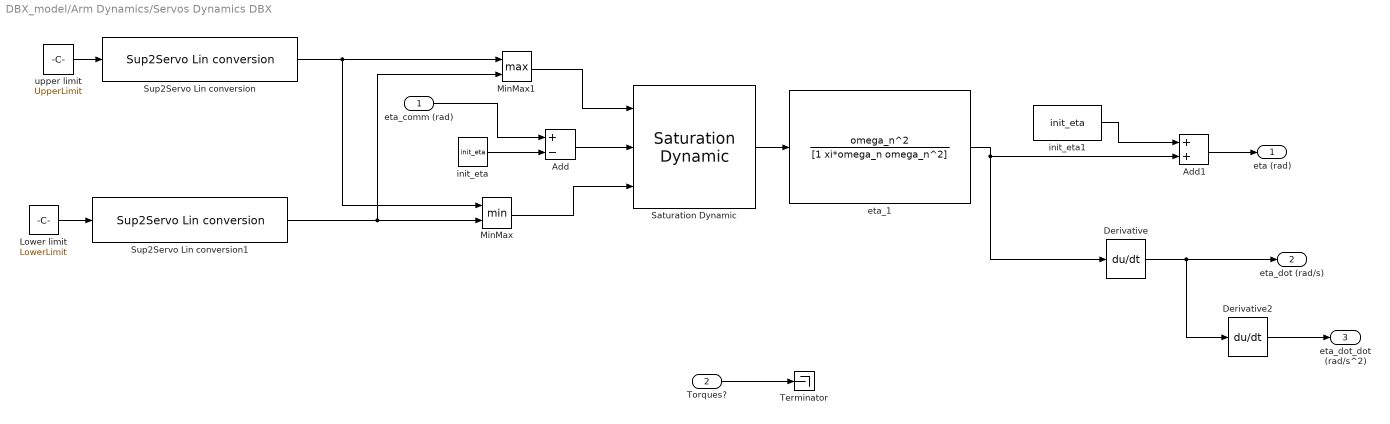
== system DBX_model/Arm Dynamics/Servos Dynamics DBX ==
  eta_comm (rad) : Inport
  Torques? : Inport  Port=2
  Add : Sum  Inputs=+-
  Add1 : Sum
  Derivative : Derivative  CoefficientInTFapproximation=derv_param
  Derivative2 : Derivative  CoefficientInTFapproximation=derv_param
  Lower limit : Constant  Value=LowerLimit
  MinMax : MinMax  Inputs=2
  MinMax1 : MinMax  Function=max  Inputs=2
  Saturation Dynamic : simulink/Discontinuities/Saturation Dynamic  OutMin=[]  OutMax=[]  OutDataTypeStr=Inherit: Same as second input  OutDataType=fixdt(1, 16)  OutScaling=2^-10  DoSatur=off
  Sup2Servo Lin conversion : DBX_model/Sup2Servo Lin conversion  Gain=Gain  Bias=Bias
  Sup2Servo Lin conversion1 : DBX_model/Sup2Servo Lin conversion  Gain=Gain  Bias=Bias
  Terminator : Terminator
  eta_1 : TransferFcn  Numerator=omega_n^2  Denominator=[1 xi*omega_n omega_n^2]
  init_eta : Constant  Value=init_eta
  init_eta1 : Constant  Value=init_eta
  upper limit : Constant  Value=UpperLimit
  eta (rad) : Outport
  eta_dot (rad/s) : Outport  Port=2
  eta_dot_dot (rad/s^2) : Outport  Port=3
  wires:
  Add1/1 -> eta (rad)/1
  init_eta1/1 -> Add1/1
  eta_1/1 -> Derivative/1, Add1/2
  Torques?/1 -> Terminator/1
  Derivative2/1 -> eta_dot_dot (rad/s^2)/1
  Derivative/1 -> Derivative2/1, eta_dot (rad/s)/1
  Add/1 -> Saturation Dynamic/2
  eta_comm (rad)/1 -> Add/1
  init_eta/1 -> Add/2
  Saturation Dynamic/1 -> eta_1/1
  upper limit/1 -> Sup2Servo Lin conversion/1
  Lower limit/1 -> Sup2Servo Lin conversion1/1
  Sup2Servo Lin conversion/1 -> MinMax1/1, MinMax/1
  Sup2Servo Lin conversion1/1 -> MinMax1/2, MinMax/2
  MinMax/1 -> Saturation Dynamic/3
  MinMax1/1 -> Saturation Dynamic/1

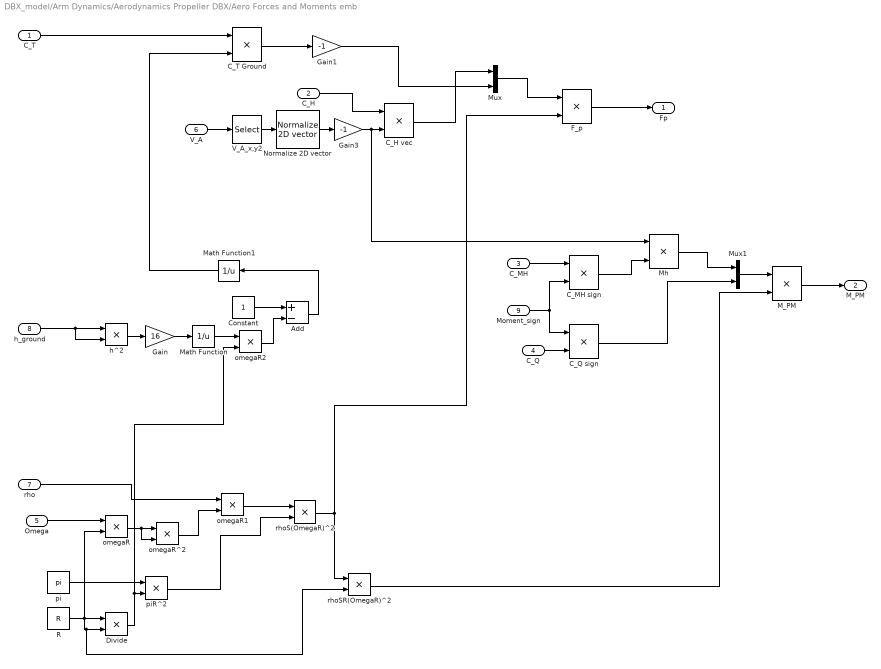
== system DBX_model/Arm Dynamics/Aerodynamics Propeller DBX/Aero Forces and Moments emb ==
  C_T : Inport
  C_H : Inport  Port=2
  C_MH : Inport  Port=3
  C_Q : Inport  Port=4
  Omega : Inport  Port=5
  V_A : Inport  Port=6
  rho : Inport  Port=7
  h_ground : Inport  Port=8
  Moment_sign : Inport  Port=9
  Add : Sum  Inputs=+-
  C_H vec : Product  Inputs=**
  C_MH sign : Product  Inputs=**
  C_Q sign : Product  Inputs=**
  C_T Ground : Product  Inputs=**
  Constant : Constant
  Divide : Product  Inputs=**
  F_p : Product  Inputs=**
  Gain : Gain  Gain=16
  Gain1 : Gain  Gain=-1
  Gain3 : Gain  Gain=-1
  M_PM : Product  Inputs=**
  Math Function : Math  Operator=reciprocal  SaturateOnIntegerOverflow=on
  Math Function1 : Math  Operator=reciprocal  SaturateOnIntegerOverflow=on
  Mh : Product  Inputs=**
  Mux : Mux  Inputs=[2,1]
  Mux1 : Mux  Inputs=[2,1]
  Normalize 2D vector : DBX_model/Normalize 2D vector
  R : Constant  Value=R
  V_A_x,y2 : Selector  IndexMode=Zero-based  InputPortWidth=3  Indices=[0,1]
  h^2 : Product  Inputs=**
  omegaR : Product  Inputs=**
  omegaR1 : Product  Inputs=**
  omegaR2 : Product  Inputs=**
  omegaR^2 : Product  Inputs=**
  pi : Constant  Value=pi
  piR^2 : Product  Inputs=**
  rhoS(OmegaR)^2 : Product  Inputs=**
  rhoSR(OmegaR)^2 : Product  Inputs=**
  Fp : Outport
  "M_PM " : Outport  Port=2
  wires:
  R/1 -> rhoSR(OmegaR)^2/2, Divide/2, omegaR/2, Divide/1
  pi/1 -> piR^2/1
  Divide/1 -> omegaR2/2, piR^2/2
  Omega/1 -> omegaR/1
  rho/1 -> omegaR1/1
  omegaR/1 -> omegaR^2/2, omegaR^2/1
  omegaR^2/1 -> omegaR1/2
  piR^2/1 -> rhoS(OmegaR)^2/2
  omegaR1/1 -> rhoS(OmegaR)^2/1
  C_T/1 -> C_T Ground/1
  h_ground/1 -> h^2/2, h^2/1
  h^2/1 -> Gain/1
  Gain/1 -> Math Function/1
  Math Function/1 -> omegaR2/1
  Constant/1 -> Add/1
  omegaR2/1 -> Add/2
  Add/1 -> Math Function1/1
  Math Function1/1 -> C_T Ground/2
  C_T Ground/1 -> Gain1/1
  V_A_x,y2/1 -> Normalize 2D vector/1
  V_A/1 -> V_A_x,y2/1
  Normalize 2D vector/1 -> Gain3/1
  Gain3/1 -> Mh/1, C_H vec/2
  C_H/1 -> C_H vec/1
  C_H vec/1 -> Mux/1
  Gain1/1 -> Mux/2
  Mux/1 -> F_p/1
  rhoS(OmegaR)^2/1 -> rhoSR(OmegaR)^2/1, F_p/2
  C_MH/1 -> C_MH sign/1
  Moment_sign/1 -> C_MH sign/2, C_Q sign/1
  C_MH sign/1 -> Mh/2
  Mh/1 -> Mux1/1
  F_p/1 -> Fp/1
  Mux1/1 -> M_PM/1
  C_Q/1 -> C_Q sign/2
  C_Q sign/1 -> Mux1/2
  rhoSR(OmegaR)^2/1 -> M_PM/2
  M_PM/1 -> "M_PM "/1

== matlab function DBX_model/Prop Coefficients MOD ==
  data: lambda input; C_T output; mu input; C_H output; C_MH output; C_Q output; sigma parameter; C_d0 parameter; a parameter; theta_0 parameter; theta_1 parameter; lambda_0_T parameter; kappa_T parameter; lambda_0_Q parameter; kappa_Q parameter
function [C_T,C_H,C_MH,C_Q] = Aero_coeff_MOD(lambda,mu, sigma, C_d0, a, theta_0, theta_1,lambda_0_T,kappa_T,lambda_0_Q,kappa_Q)

C_T = sigma*a/4*(theta_0*(2/3+mu^2) +theta_1/2*(1+mu^2) -  kappa_T*(lambda-lambda_0_T)^2 );
C_Q =    +sigma*a/4*( 2/3*theta_0 -  kappa_Q*(lambda-lambda_0_Q)^2  + theta_1/2)*kappa_Q*(lambda-lambda_0_Q)^2 + sigma*C_d0/8*(1+mu^2);   % Always positive!!!


C_H= sigma*a/4*mu*lambda*(theta_0+theta_1/2) + sigma*C_d0/4*mu; 
C_MH= sigma*a/4*( 2/3*theta_0*mu-1/2*lambda*mu+theta_1*mu/2  );

== matlab function DBX_model/Arm Dynamics/Aerodynamics Propeller DBX/Prop Coefficients MOD ==
  data: lambda input; C_T output; mu input; C_H output; C_MH output; C_Q output; sigma parameter; C_d0 parameter; a parameter; theta_0 parameter; theta_1 parameter; lambda_0_T parameter; kappa_T parameter; lambda_0_Q parameter; kappa_Q parameter
function [C_T,C_H,C_MH,C_Q] = Aero_coeff_MOD(lambda,mu, sigma, C_d0, a, theta_0, theta_1,lambda_0_T,kappa_T,lambda_0_Q,kappa_Q)

C_T = sigma*a/4*(theta_0*(2/3+mu^2) +theta_1/2*(1+mu^2) -  kappa_T*(lambda-lambda_0_T)^2 );
C_Q =    +sigma*a/4*( 2/3*theta_0 -  kappa_Q*(lambda-lambda_0_Q)^2  + theta_1/2)*kappa_Q*(lambda-lambda_0_Q)^2 + sigma*C_d0/8*(1+mu^2);   % Always positive!!!


C_H= sigma*a/4*mu*lambda*(theta_0+theta_1/2) + sigma*C_d0/4*mu; 
C_MH= sigma*a/4*( 2/3*theta_0*mu-1/2*lambda*mu+theta_1*mu/2  );

== matlab function DBX_model/Arm Dynamics/ESC+Motor Dynamcis DBX/Motor_efficiency ==
  data: Amps input; eta output
function eta = eta_motor(Amps)


eta = max(0.01,0.8-exp(-0.2*Amps));

== matlab function DBX_model/Gravity Force and Moment ==
  data: q input; F_g_b output; M_g_b output; mass input; CG input; g parameter
function [F_g_b,M_g_b]   = Grav_Forces_and_Mom( q,mass,CG, g)

Prod=HamiltonProduct([q(1);-q(2);-q(3);-q(4)],HamiltonProduct([0;0;0;mass*g],[q(1);q(2);q(3);q(4)]) ); % q* . g .q

F_g_b= Prod(2:4);
M_g_b=cross(CG,F_g_b);


function Product= HamiltonProduct( a,b )

Product=[ a(1)*b(1)-a(2)*b(2)-a(3)*b(3)-a(4)*b(4) ; a(1)*b(2)+a(2)*b(1)+a(3)*b(4)-a(4)*b(3)  ; a(1)*b(3)-a(2)*b(4)+a(3)*b(1)+a(4)*b(2)  ; a(1)*b(4)+a(2)*b(3)-a(3)*b(2)+a(4)*b(1) ];

== matlab function DBX_model/ISA ==
  data: altitude input; rho output; T output; Ps output; a output
function [rho,T,Ps,a]= ISA_atmos(altitude)


    rho0 = 1.225; tfac = 1 - 6.5e-3/288.15*altitude;
    T = 288.15*tfac; if (altitude >= 11000) T = 216.65; end;
    rho = rho0*(tfac.^4.2586);
    Ps = 287*rho*T;
    a=sqrt(1.4*287*T);
    
end

== matlab function DBX_model/Arm Dynamics/Arms Kinematics DBX/DCM Arm ==
  data: arm_no input; eta input; T_Fb_FA output
function T_Fb_FA = DCM_Arm(arm_no,eta)
if arm_no==1 || arm_no==2
    T_Fb_FA = [ cos(eta),0,-sin(eta);
                    0,1,0;
                sin(eta),0,cos(eta)];
elseif arm_no==3 
    T_Fb_FA = [1,0,0;
                0,cos(eta),sin(eta);
                0,-sin(eta),cos(eta)];
else
    error('That is not right: Chose a right arm'); 
end

== matlab function DBX_model/Prop Coefficients ==
  data: lambda input; C_T output; mu input; C_H output; C_MH output; C_Q output; sigma parameter; C_d0 parameter; a parameter; theta_0 parameter; theta_1 parameter
function [C_T,C_H,C_MH,C_Q] = Aero_coeff(lambda,mu, sigma, C_d0, a, theta_0, theta_1)

C_T = sigma*a/4*(theta_0*(2/3+mu^2) +theta_1/2*(1+mu^2) -  lambda );
C_Q =    +sigma*a/4*( 2/3*theta_0 - lambda + theta_1/2)*lambda + sigma*C_d0/8*(1+mu^2);   % Always positive!!!


C_H= sigma*a/4*mu*lambda*(theta_0+theta_1/2) + sigma*C_d0/4*mu; 
C_MH= sigma*a/4*( 2/3*theta_0*mu-1/2*lambda*mu+theta_1*mu/2  );

== matlab function DBX_model/Ground  model/Ground model logic and Forces and moments ==
  data: Xe input; Vb input; q input; omega_b input; F_gr_b output; M_gr_b output; mass input; g parameter; Arm1 input; Arm2 input; Arm3 input
function [F_gr_b,M_gr_b]   = Gorund_Forces_and_Mom( Xe,Vb,q,omega_b,mass, g, Arm1,Arm2,Arm3)

F_gr_b=zeros(3,1);
M_gr_b=zeros(3,1);


% Arm 1
Prod=HamiltonProduct([q(1);q(2);q(3);q(4)],HamiltonProduct([0;Arm1],[q(1);-q(2);-q(3);-q(4)]) ); % q . Arm .q*: From body to earth axes
h_arm1 = Xe(3) + Prod(2:4);
% Arm 2
Prod=HamiltonProduct([q(1);q(2);q(3);q(4)],HamiltonProduct([0;Arm2],[q(1);-q(2);-q(3);-q(4)]) ); % q . Arm .q*: From body to earth axes
h_arm2 = Xe(3) + Prod(2:4);
% Arm 3
Prod=HamiltonProduct([q(1);q(2);q(3);q(4)],HamiltonProduct([0;Arm3],[q(1);-q(2);-q(3);-q(4)]) ); % q . Arm .q*: From body to earth axes
h_arm3 = Xe(3) + Prod(2:4);


min_h = max([Xe(3),h_arm1(3),h_arm2(3),h_arm3(3)]);
if min_h >=-0.01  &&  min_h <= 0  && Vb(3)>0
    Prod=HamiltonProduct([q(1);-q(2);-q(3);-q(4)],HamiltonProduct([0;0;0;-mass*g],[q(1);q(2);q(3);q(4)]) ); % q* . g .q: From earth to Body axes
    F_gr_b= Prod(2:4);
    %Friction forces
    F_gr_b = F_gr_b - 5*Vb;
    
elseif min_h >=-0.01  &&  min_h >0
    Prod=HamiltonProduct([q(1);-q(2);-q(3);-q(4)],HamiltonProduct([0;0;0; -5000*min_h ],[q(1);q(2);q(3);q(4)]) ); % q* . g .q: From earth to Body axes
    F_gr_b =  Prod(2:4);
    %Friction forces
    F_gr_b = F_gr_b - 250*Vb;
else
    F_gr_b=zeros(3,1);

end


% Moments
Prod=HamiltonProduct([q(1);-q(2);-q(3);-q(4)],HamiltonProduct([0;0;0;-mass*g],[q(1);q(2);q(3);q(4)]) ); % q* . g .q: From earth to Body axes
F_g = Prod(2:4);
if min_h >=-0.01
    if h_arm1(3)>max(h_arm2(3),h_arm3(3))+0.01
        M_gr_b=cross(Arm1,F_g);
    elseif h_arm1(3)<max(h_arm2(3),h_arm3(3))-0.01  && h_arm2(3)>h_arm3(3)+0.01
        M_gr_b=cross(Arm2,F_g);
    elseif h_arm1(3)<max(h_arm2(3),h_arm3(3))-0.01  && h_arm3(3)>h_arm2(3)+0.01
        M_gr_b=cross(Arm3,F_g);
    elseif h_arm1(3)<max(h_arm2(3),h_arm3(3))-0.01  && abs( h_arm3(3)-h_arm2(3) )<=0.01
        M_gr_b=cross( sum([Arm2,Arm3],2)/2,F_g);
        
    else
        M_gr_b=zeros(3,1);
    end
    M_gr_b = M_gr_b -20*omega_b;
else
    M_gr_b=zeros(3,1);
end



function Product= HamiltonProduct( a,b )

Product=[ a(1)*b(1)-a(2)*b(2)-a(3)*b(3)-a(4)*b(4) ; a(1)*b(2)+a(2)*b(1)+a(3)*b(4)-a(4)*b(3)  ; a(1)*b(3)-a(2)*b(4)+a(3)*b(1)+a(4)*b(2)  ; a(1)*b(4)+a(2)*b(3)-a(3)*b(2)+a(4)*b(1) ];
